simulink model "Resistance_Forces_ABB_FORMULA_Drive_Cycle"  (R2015a)
settings: Solver=ode45  StartTime=0.0  StopTime=maxtime  RelTol=1e-3
values from neighbouring files (symbols this model uses):
  A = 1.8585    [Drive_Cycle_Read_Script.m]
  Cd = 0.9    [Drive_Cycle_Read_Script.m]
  Crr = 0.015    [Drive_Cycle_Read_Script.m]
  GVM = 900    [Drive_Cycle_Read_Script.m]
  GVW = GVM*g    (= 8829)    [Drive_Cycle_Read_Script.m]
  rho = 1.225    [Drive_Cycle_Read_Script.m]
  Rw = 0.2286    [Drive_Cycle_Read_Script.m]
settings Model: Creator=Koustubh  LastModifiedBy=Koustubh

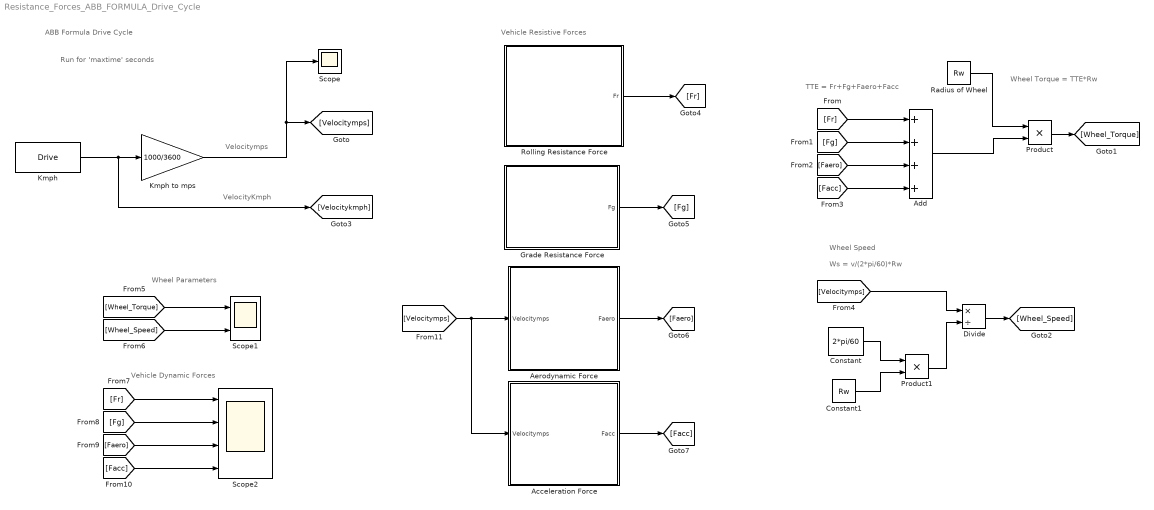
== system Resistance_Forces_ABB_FORMULA_Drive_Cycle ==
  note: Vehicle Dynamic Forces
  note: Wheel Parameters
  note: Vehicle Resistive Forces
  note: Ws = v/(2*pi/60)*Rw
  note: Wheel Speed
  note: TTE = Fr+Fg+Faero+Facc
  note: Wheel Torque = TTE*Rw
  note: Run for 'maxtime' seconds
  note: VelocityKmph
  note: Velocitymps
  note: ABB Formula Drive Cycle
  Acceleration Force : Subsystem
      mask Display: image(imread('F:\Internships\Decibels Lab\Docs\Week-2\Facc.jpg'))
  Add : Sum  Inputs=++++
  Aerodynamic Force : Subsystem
      mask Display: image(imread('F:\Internships\Decibels Lab\Docs\Week-2\Faero.png'))
  Constant : Constant  Value=2*pi/60
  Constant1 : Constant  Value=Rw
  Divide : Product  Inputs=*/
  Grade Resistance Force : Subsystem
      mask Display: image(imread('F:\Internships\Decibels Lab\Docs\Week-2\Fg.jpg'))
  Kmph : FromWorkspace  VariableName=Drive  SampleTime=0
  Kmph to mps : Gain  Gain=1000/3600
  Product : Product
  Product1 : Product
  Radius of Wheel : Constant  Value=Rw
  Rolling Resistance Force : Subsystem
      mask Display: image(imread('F:\Internships\Decibels Lab\Docs\Week-2\Fr.jpg'))
  Scope : Scope
  Scope1 : Scope  NumInputPorts=2
      settings: YMin=-5~-5  YMax=5~5
  Scope2 : Scope  NumInputPorts=4
      settings: YMin=-5~-5~-5~-5  YMax=5~5~5~5  SaveName=ScopeData4
  wires:
  Kmph/1 -> [Velocitykmph], Kmph to mps/1
  Kmph to mps/1 -> Scope/1, [Velocitymps]
  [Fr] -> Add/1
  [Fg] -> Add/2
  [Faero] -> Add/3
  [Facc] -> Add/4
  Radius of Wheel/1 -> Product/1
  Add/1 -> Product/2
  Product/1 -> [Wheel_Torque]
  Constant/1 -> Product1/1
  Constant1/1 -> Product1/2
  Product1/1 -> Divide/2
  [Velocitymps] -> Divide/1
  Divide/1 -> [Wheel_Speed]
  [Wheel_Speed] -> Scope1/2
  [Fr] -> Scope2/1
  [Fg] -> Scope2/2
  [Faero] -> Scope2/3
  [Facc] -> Scope2/4
  [Velocitymps] -> Acceleration Force/1(Velocitymps), Aerodynamic Force/1(Velocitymps)
  Acceleration Force/1(Facc) -> [Facc]
  Aerodynamic Force/1(Faero) -> [Faero]
  Grade Resistance Force/1(Fg) -> [Fg]
  Rolling Resistance Force/1(Fr) -> [Fr]
  [Wheel_Torque] -> Scope1/1

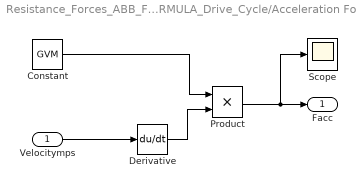
== system Resistance_Forces_ABB_FORMULA_Drive_Cycle/Acceleration Force ==
  Velocitymps : Inport
  Constant : Constant  Value=GVM
  Derivative : Derivative
  Product : Product
  Scope : Scope
      settings: SaveName=ScopeData5
  Facc : Outport
  wires:
  Derivative/1 -> Product/2
  Constant/1 -> Product/1
  Velocitymps/1 -> Derivative/1
  Product/1 -> Facc/1, Scope/1

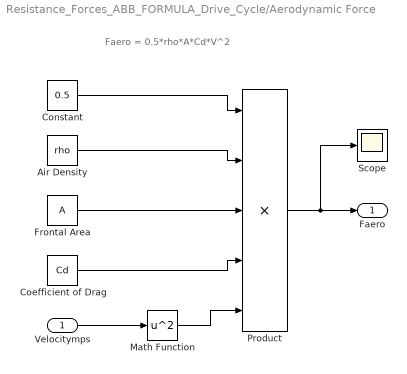
== system Resistance_Forces_ABB_FORMULA_Drive_Cycle/Aerodynamic Force ==
  note: Faero = 0.5*rho*A*Cd*V^2
  Velocitymps : Inport
  Air Density : Constant  Value=rho
  Coefficient of Drag : Constant  Value=Cd
  Constant : Constant  Value=0.5
  Frontal Area : Constant  Value=A
  Math Function : Math  Operator=square  SaturateOnIntegerOverflow=on
  Product : Product  Inputs=5
  Scope : Scope
      settings: SaveName=ScopeData3
  Faero : Outport
  wires:
  Coefficient of Drag/1 -> Product/4
  Constant/1 -> Product/1
  Frontal Area/1 -> Product/3
  Velocitymps/1 -> Math Function/1
  Air Density/1 -> Product/2
  Math Function/1 -> Product/5
  Product/1 -> Faero/1, Scope/1

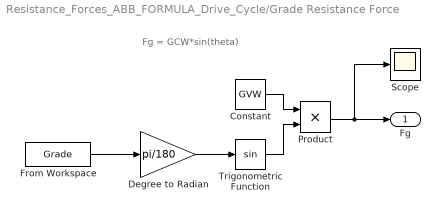
== system Resistance_Forces_ABB_FORMULA_Drive_Cycle/Grade Resistance Force ==
  note: Fg = GCW*sin(theta)
  Constant : Constant  Value=GVW
  Degree to Radian : Gain  Gain=pi/180
  From Workspace : FromWorkspace  VariableName=Grade  SampleTime=0
  Product : Product
  Scope : Scope
      settings: SaveName=ScopeData2
  Trigonometric Function : Trigonometry
  Fg : Outport
  wires:
  Degree to Radian/1 -> Trigonometric Function/1
  From Workspace/1 -> Degree to Radian/1
  Constant/1 -> Product/1
  Trigonometric Function/1 -> Product/2
  Product/1 -> Fg/1, Scope/1

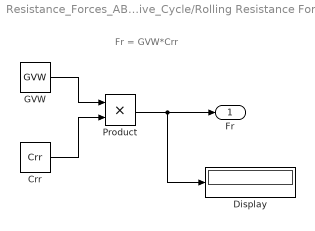
== system Resistance_Forces_ABB_FORMULA_Drive_Cycle/Rolling Resistance Force ==
  note: Fr = GVW*Crr
  Crr : Constant  Value=Crr
  Display : Display
  GVW : Constant  Value=GVW
  Product : Product
  Fr : Outport
  wires:
  Crr/1 -> Product/2
  Product/1 -> Fr/1, Display/1
  GVW/1 -> Product/1
